simulink model "simulink_rc_devre1"  (R2013a)
settings: Solver=ode45  StartTime=0.0  StopTime=10.0  RelTol=1e-3
undefined symbols (not defined in the file or in its folder): s
settings Model: Creator=alper pc  LastModifiedBy=alper pc

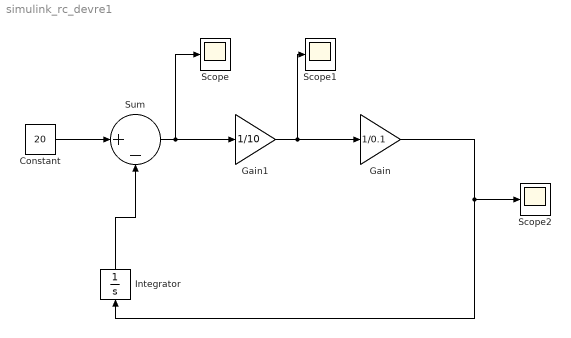
== system simulink_rc_devre1 ==
  Constant : Constant  Value=20
  Gain : Gain  Gain=1/0.1
  Gain1 : Gain  Gain=1/10
  Integrator : Integrator  InitialCondition=s
  Scope : Scope
  Scope1 : Scope
  Scope2 : Scope
      settings: SaveName=ScopeData2
  Sum : Sum  Inputs=|+-
  wires:
  Constant/1 -> Sum/1
  Sum/1 -> Scope/1, Gain1/1
  Gain1/1 -> Scope1/1, Gain/1
  Integrator/1 -> Sum/2
  Gain/1 -> Integrator/1, Scope2/1
